simulink model "Seq_demo1"  (R2025b)
settings: Solver=FixedStepAuto  StartTime=0.0  StopTime=Inf  RelTol=1e-3
libraries: SignalEditorBlockLib x1
settings Model: Creator=Soochan Kim  LastModifiedBy=Soochan Kim

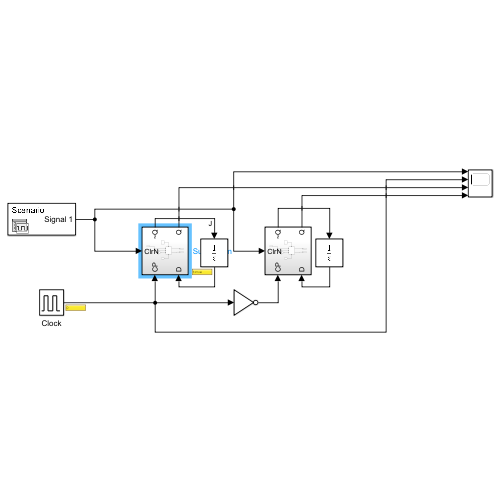
[thumbnail: Simulink's stored preview of the top-level diagram]
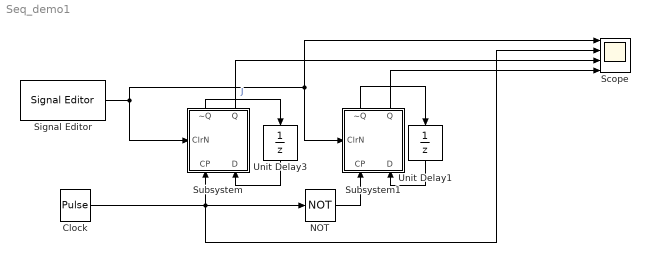
== system Seq_demo1 ==
  Clock : DiscretePulseGenerator  PulseType=Time based  PulseWidth=50  PhaseDelay=1
  NOT : Logic  Operator=NOT  IconShape=distinctive  AllPortsSameDT=off  OutDataTypeStr=boolean
  Scope : Scope  NumInputPorts=4
      settings: ActiveDisplayYMinimum=-0.12499999999999997  ActiveDisplayYMaximum=1.125
  Signal Editor : SignalEditorBlockLib/Signal Editor  FileName=ClrN.mat  ActiveScenario=Scenario  ActiveSignal=Signal 1  IsBus=off  OutputBusObjectStr=Bus: BusObject  SampleTime=0  ZeroCross=off  OutputAfterFinalValue=Setting to zero  Unit=inherit  PreserveSignalName=on  ApplySigPropsToAllScenarios=on  ApplySigPropsToAllSignals=off  SignalPropertySource=Dialog parameters
  Subsystem : Subsystem
      settings: PortSchema="{\"entries\":[{\"content\":{\"sides\":[{\"content\":{\"connectorIds\":[\"In1\",\"In2\"]},\"type\":\"ConnectorPlacement.EquallySpacedRectSide\",\"uuid\":\"1850862e-0981-4c6a-92eb-2c432b23f3fe\"},{\"content\":{\"connectorIds\":[\"Out1\",\"Out2\"],\"side\":\"RIGHT\"},\"type\":\"ConnectorPlacement.EquallySpacedRectSide\",\"uuid\":\"bcd843d6-a758-4620-a6e3-e1caee8a013e\"},{\"content\":{\"side\":\"TOP\"},\"type\":\"ConnectorPlacement.EquallySpacedRectSide\",\"uuid\":\"251bd3d3-3218-4c98-8967-89bf8dc84763\"},{\"content\":{\"connectorIds\":[\"In3\"],\"side\":\"BOTTOM\"},\"type\":\"ConnectorPlacement.EquallySpacedRectSide\",\"uuid\":\"25d92a0a-f581-4d72-9648-6406fc3ab92b\"}]},\"type\":\"ConnectorPlacement.EquallySpacedConnector\",\"uuid\":\"0a81c46f-fac3-4488-9c91-54b3c40e9e1d\"}],\"packageUris\":[\"http://schema.mathworks.com/mf0/Connector/R2020b\"],\"version\":\"1.0\"}"
  Subsystem1 : Subsystem
      settings: PortSchema="{\"entries\":[{\"content\":{\"sides\":[{\"content\":{\"connectorIds\":[\"In1\",\"In2\"]},\"type\":\"ConnectorPlacement.EquallySpacedRectSide\",\"uuid\":\"1850862e-0981-4c6a-92eb-2c432b23f3fe\"},{\"content\":{\"connectorIds\":[\"Out1\",\"Out2\"],\"side\":\"RIGHT\"},\"type\":\"ConnectorPlacement.EquallySpacedRectSide\",\"uuid\":\"bcd843d6-a758-4620-a6e3-e1caee8a013e\"},{\"content\":{\"side\":\"TOP\"},\"type\":\"ConnectorPlacement.EquallySpacedRectSide\",\"uuid\":\"251bd3d3-3218-4c98-8967-89bf8dc84763\"},{\"content\":{\"connectorIds\":[\"In3\"],\"side\":\"BOTTOM\"},\"type\":\"ConnectorPlacement.EquallySpacedRectSide\",\"uuid\":\"25d92a0a-f581-4d72-9648-6406fc3ab92b\"}]},\"type\":\"ConnectorPlacement.EquallySpacedConnector\",\"uuid\":\"0a81c46f-fac3-4488-9c91-54b3c40e9e1d\"}],\"packageUris\":[\"http://schema.mathworks.com/mf0/Connector/R2020b\"],\"version\":\"1.0\"}"
  Unit Delay1 : UnitDelay  SampleTime=0.001  HasFrameUpgradeWarning=on
  Unit Delay3 : UnitDelay  SampleTime=0.001  HasFrameUpgradeWarning=on
  wires:
  Subsystem/2(~Q) -> Unit Delay3/1  "J"
  NOT/1 -> Subsystem1/2(CP)
  Clock/1 -> Subsystem/2(CP), Scope/2, NOT/1
  Signal Editor/1 -> Subsystem/3(ClrN), Subsystem1/3(ClrN), Scope/1
  Subsystem1/2(~Q) -> Unit Delay1/1
  Unit Delay3/1 -> Subsystem/1(D)
  Unit Delay1/1 -> Subsystem1/1(D)
  Subsystem/1(Q) -> Scope/3
  Subsystem1/1(Q) -> Scope/4

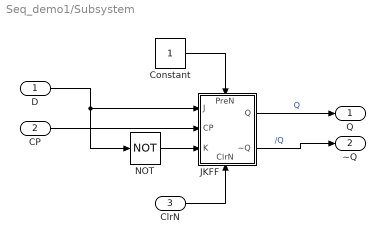
== system Seq_demo1/Subsystem ==
  D : Inport
  CP : Inport  Port=2
  ClrN : Inport  Port=3
  Constant : Constant
  JKFF : Subsystem
      settings: PortSchema="{\"entries\":[{\"content\":{\"sides\":[{\"content\":{\"connectorIds\":[\"In1\",\"In2\",\"In3\"]},\"type\":\"ConnectorPlacement.EquallySpacedRectSide\",\"uuid\":\"ca5f62ac-258f-4342-b449-d4588bf63b40\"},{\"content\":{\"connectorIds\":[\"Out1\",\"Out2\"],\"side\":\"RIGHT\"},\"type\":\"ConnectorPlacement.EquallySpacedRectSide\",\"uuid\":\"b147f298-1794-4db6-92d9-78f3dcdc57bc\"},{\"content\":{\"connectorIds\":[\"In4\"],\"side\":\"TOP\"},\"type\":\"ConnectorPlacement.EquallySpacedRectSide\",\"uuid\":\"71d3f859-1ac9-4aca-bc8d-fdbc7575d1a1\"},{\"content\":{\"connectorIds\":[\"In5\"],\"side\":\"BOTTOM\"},\"type\":\"ConnectorPlacement.EquallySpacedRectSide\",\"uuid\":\"d95374ea-5ccb-478e-ae62-65b01aae921e\"}]},\"type\":\"ConnectorPlacement.EquallySpacedConnector\",\"uuid\":\"23ee79f5-4ac2-4c37-9e5e-b94b9950e040\"}],\"packageUris\":[\"http://schema.mathworks.com/mf0/Connector/R2020b\"],\"version\":\"1.0\"}"
  NOT : Logic  Operator=NOT  IconShape=distinctive  AllPortsSameDT=off  OutDataTypeStr=boolean
  Q : Outport
  ~Q : Outport  Port=2
  wires:
  NOT/1 -> JKFF/3(K)
  D/1 -> NOT/1, JKFF/1(J)
  JKFF/2(~Q) -> ~Q/1  "/Q"
  CP/1 -> JKFF/2(CP)
  JKFF/1(Q) -> Q/1  "Q"
  Constant/1 -> JKFF/4(PreN)
  ClrN/1 -> JKFF/5(ClrN)

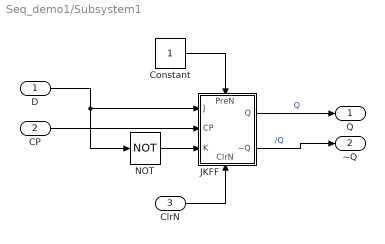
== system Seq_demo1/Subsystem1 ==
  D : Inport
  CP : Inport  Port=2
  ClrN : Inport  Port=3
  Constant : Constant
  JKFF : Subsystem
      settings: PortSchema="{\"entries\":[{\"content\":{\"sides\":[{\"content\":{\"connectorIds\":[\"In1\",\"In2\",\"In3\"]},\"type\":\"ConnectorPlacement.EquallySpacedRectSide\",\"uuid\":\"ca5f62ac-258f-4342-b449-d4588bf63b40\"},{\"content\":{\"connectorIds\":[\"Out1\",\"Out2\"],\"side\":\"RIGHT\"},\"type\":\"ConnectorPlacement.EquallySpacedRectSide\",\"uuid\":\"b147f298-1794-4db6-92d9-78f3dcdc57bc\"},{\"content\":{\"connectorIds\":[\"In4\"],\"side\":\"TOP\"},\"type\":\"ConnectorPlacement.EquallySpacedRectSide\",\"uuid\":\"71d3f859-1ac9-4aca-bc8d-fdbc7575d1a1\"},{\"content\":{\"connectorIds\":[\"In5\"],\"side\":\"BOTTOM\"},\"type\":\"ConnectorPlacement.EquallySpacedRectSide\",\"uuid\":\"d95374ea-5ccb-478e-ae62-65b01aae921e\"}]},\"type\":\"ConnectorPlacement.EquallySpacedConnector\",\"uuid\":\"23ee79f5-4ac2-4c37-9e5e-b94b9950e040\"}],\"packageUris\":[\"http://schema.mathworks.com/mf0/Connector/R2020b\"],\"version\":\"1.0\"}"
  NOT : Logic  Operator=NOT  IconShape=distinctive  AllPortsSameDT=off  OutDataTypeStr=boolean
  Q : Outport
  ~Q : Outport  Port=2
  wires:
  NOT/1 -> JKFF/3(K)
  D/1 -> NOT/1, JKFF/1(J)
  JKFF/2(~Q) -> ~Q/1  "/Q"
  CP/1 -> JKFF/2(CP)
  JKFF/1(Q) -> Q/1  "Q"
  Constant/1 -> JKFF/4(PreN)
  ClrN/1 -> JKFF/5(ClrN)

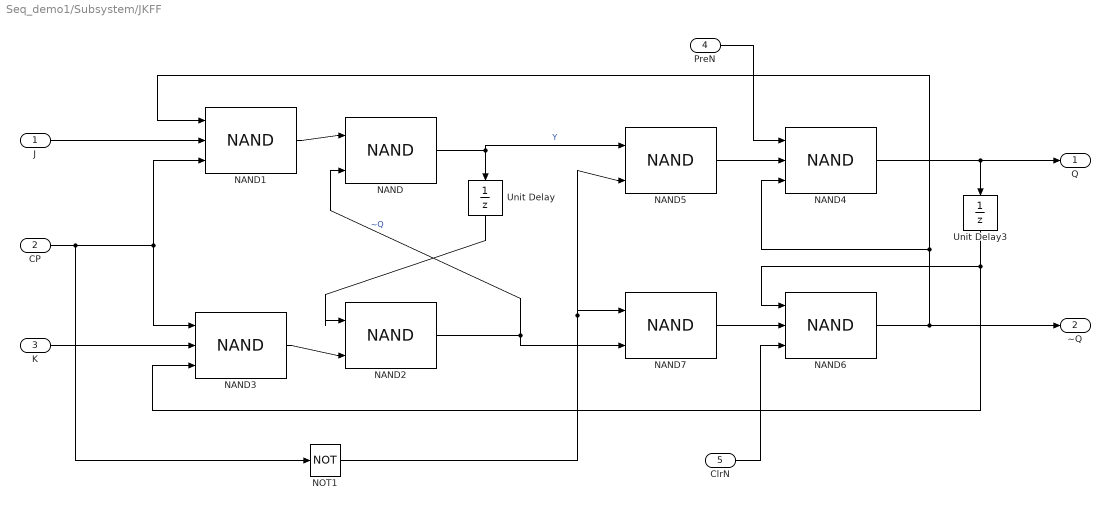
== system Seq_demo1/Subsystem/JKFF ==
  J : Inport
  CP : Inport  Port=2
  K : Inport  Port=3
  PreN : Inport  Port=4
  ClrN : Inport  Port=5
  NAND{,2,5,7} (4 alike) : Logic  Operator=NAND  IconShape=distinctive  AllPortsSameDT=off  OutDataTypeStr=boolean
  NAND{1,3..4,6} (4 alike) : Logic  Operator=NAND  Inputs=3  IconShape=distinctive  AllPortsSameDT=off  OutDataTypeStr=boolean
  NOT1 : Logic  Operator=NOT  IconShape=distinctive  AllPortsSameDT=off  OutDataTypeStr=boolean
  Unit Delay : UnitDelay  SampleTime=0.001  HasFrameUpgradeWarning=on
  Unit Delay3 : UnitDelay  SampleTime=-1  HasFrameUpgradeWarning=on
  Q : Outport
  ~Q : Outport  Port=2
  wires:
  NAND/1 -> Unit Delay/1, NAND5/1  "Y"
  NAND2/1 -> NAND/2, NAND7/2  "~Q"
  Unit Delay/1 -> NAND2/1
  K/1 -> NAND3/2
  NAND1/1 -> NAND/1
  NAND3/1 -> NAND2/2
  J/1 -> NAND1/2
  NAND6/1 -> NAND1/1, NAND4/3, ~Q/1
  Unit Delay3/1 -> NAND3/3, NAND6/1
  NAND7/1 -> NAND6/2
  NAND4/1 -> Unit Delay3/1, Q/1
  CP/1 -> NAND1/3, NAND3/1, NOT1/1
  NOT1/1 -> NAND5/2, NAND7/1
  NAND5/1 -> NAND4/2
  PreN/1 -> NAND4/1
  ClrN/1 -> NAND6/3

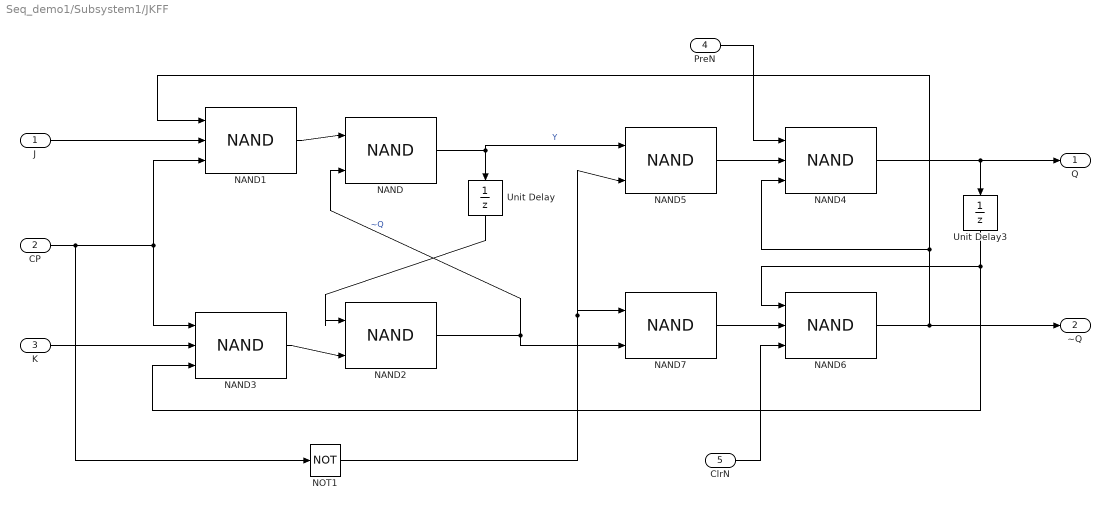
== system Seq_demo1/Subsystem1/JKFF ==
  J : Inport
  CP : Inport  Port=2
  K : Inport  Port=3
  PreN : Inport  Port=4
  ClrN : Inport  Port=5
  NAND{,2,5,7} (4 alike) : Logic  Operator=NAND  IconShape=distinctive  AllPortsSameDT=off  OutDataTypeStr=boolean
  NAND{1,3..4,6} (4 alike) : Logic  Operator=NAND  Inputs=3  IconShape=distinctive  AllPortsSameDT=off  OutDataTypeStr=boolean
  NOT1 : Logic  Operator=NOT  IconShape=distinctive  AllPortsSameDT=off  OutDataTypeStr=boolean
  Unit Delay : UnitDelay  SampleTime=0.001  HasFrameUpgradeWarning=on
  Unit Delay3 : UnitDelay  SampleTime=-1  HasFrameUpgradeWarning=on
  Q : Outport
  ~Q : Outport  Port=2
  wires:
  NAND/1 -> Unit Delay/1, NAND5/1  "Y"
  NAND2/1 -> NAND/2, NAND7/2  "~Q"
  Unit Delay/1 -> NAND2/1
  K/1 -> NAND3/2
  NAND1/1 -> NAND/1
  NAND3/1 -> NAND2/2
  J/1 -> NAND1/2
  NAND6/1 -> NAND1/1, NAND4/3, ~Q/1
  Unit Delay3/1 -> NAND3/3, NAND6/1
  NAND7/1 -> NAND6/2
  NAND4/1 -> Unit Delay3/1, Q/1
  CP/1 -> NAND1/3, NAND3/1, NOT1/1
  NOT1/1 -> NAND5/2, NAND7/1
  NAND5/1 -> NAND4/2
  PreN/1 -> NAND4/1
  ClrN/1 -> NAND6/3
